simulink model "simulation_19a_lissajous"  (R2019b)
settings: Solver=VariableStepAuto  StartTime=0.0  StopTime=60  FixedStep=1e-1  RelTol=1e-3
undefined symbols (not defined in the file or in its folder): a1, a2, int_a_err, Ke, Kk, q_0
settings Model: Creator=Mathew  LastModifiedBy=Mardok
settings SFSimCC: CustomCodeUndefinedFunction=UseInterfaceOnly

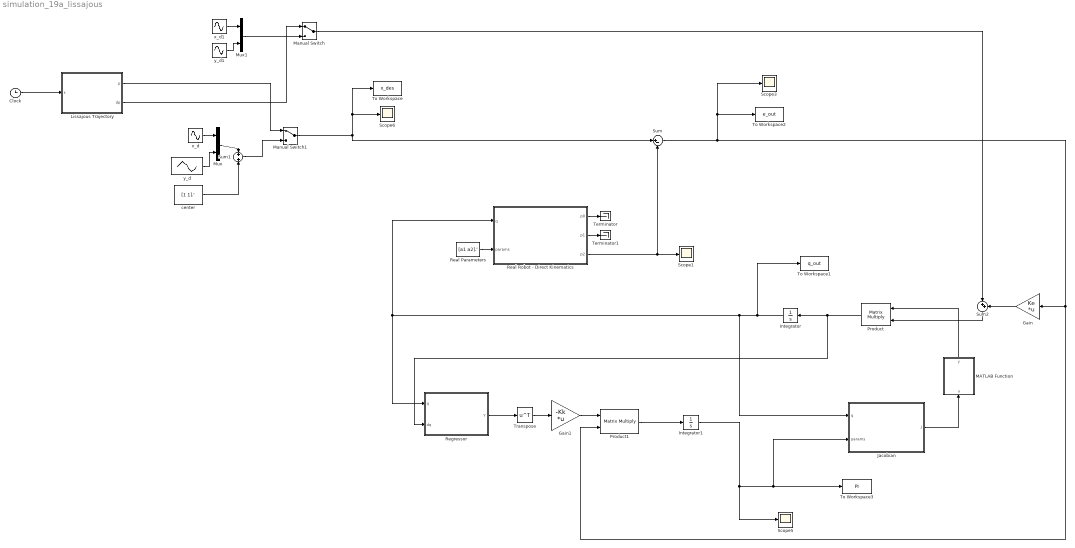
== system simulation_19a_lissajous ==
  Clock : Clock
  Gain : Gain  Gain=Ke  Multiplication=Matrix(K*u)
  Gain1 : Gain  Gain=-Kk  Multiplication=Matrix(K*u)
  Integrator : Integrator  InitialCondition=q_0
  Integrator1 : Integrator  InitialCondition=int_a_err*[a1 a2].'
  "Jacobian " : MATLAB Function  TreatAsAtomicUnit=on
  Lissajous Trajectory : MATLAB Function  TreatAsAtomicUnit=on
  MATLAB Function : MATLAB Function  TreatAsAtomicUnit=on
  Manual Switch : ManualSwitch
  Manual Switch1 : ManualSwitch
  Mux : Mux  Inputs=2
  Mux1 : Mux  Inputs=2
  Product : Product  Multiplication=Matrix(*)
  Product1 : Product  Multiplication=Matrix(*)
  Real Parameters : Constant  Value=[a1 a2].'
  Real Robot - Direct Kinematics : MATLAB Function  TreatAsAtomicUnit=on
  Regressor : MATLAB Function  TreatAsAtomicUnit=on
  Scope{1,3,5..6} (4 alike) : Scope
  Sum : Sum  Inputs=|+-
  Sum1 : Sum
  Sum2 : Sum  Inputs=|++
  Terminator : Terminator
  Terminator1 : Terminator
  To Workspace : ToWorkspace  VariableName=x_des  SaveFormat=Timeseries  SampleTime=-1
  To Workspace1 : ToWorkspace  VariableName=q_out  SaveFormat=Timeseries  SampleTime=-1
  To Workspace2 : ToWorkspace  VariableName=e_out  SaveFormat=Timeseries  SampleTime=-1
  To Workspace3 : ToWorkspace  VariableName=PI  SaveFormat=Timeseries  SampleTime=-1
  Transpose : Math  Operator=transpose  SaturateOnIntegerOverflow=on
  center : Constant  Value=[1 1].'
  x_d : Sin  Amplitude=0.25  SampleTime=0
  x_d1 : Sin  Amplitude=0.25  Phase=pi/2  SampleTime=0
  y_d : Sin  Amplitude=0.25  Phase=pi/2  SampleTime=0
  y_d1 : Sin  Amplitude=-0.25  SampleTime=0
  wires:
  Real Robot - Direct Kinematics/1(p0) -> Terminator/1
  Real Robot - Direct Kinematics/2(p1) -> Terminator1/1
  x_d/1 -> Mux/1
  y_d/1 -> Mux/2
  Manual Switch1/1 -> To Workspace/1, Scope6/1, Sum/1
  Real Robot - Direct Kinematics/3(p2) -> Scope1/1, Sum/2
  Sum/1 -> To Workspace2/1, Scope3/1, Product1/2, Gain/1
  Gain/1 -> Sum2/2
  Sum2/1 -> Product/2
  "Jacobian "/1(J) -> MATLAB Function/1(u)
  MATLAB Function/1(y) -> Product/1
  Product/1 -> Integrator/1, Regressor/2(dq)
  Integrator/1 -> To Workspace1/1, Real Robot - Direct Kinematics/1(q), Regressor/1(q), "Jacobian "/1(q)
  Regressor/1(Y) -> Transpose/1
  Transpose/1 -> Gain1/1
  Real Parameters/1 -> Real Robot - Direct Kinematics/2(params)
  Gain1/1 -> Product1/1
  Product1/1 -> Integrator1/1
  Integrator1/1 -> Scope5/1, To Workspace3/1, "Jacobian "/2(params)
  center/1 -> Sum1/2
  Mux/1 -> Sum1/1
  Manual Switch/1 -> Sum2/1
  y_d1/1 -> Mux1/2
  x_d1/1 -> Mux1/1
  Clock/1 -> Lissajous Trajectory/1(t)
  Mux1/1 -> Manual Switch/2
  Sum1/1 -> Manual Switch1/2
  Lissajous Trajectory/1(p) -> Manual Switch1/1
  Lissajous Trajectory/2(dp) -> Manual Switch/1

== matlab function simulation_19a_lissajous/Jacobian  ==
  data: q input; J output; params input
function J = J_fun( q , params)

q1 = q(1);
q2 = q(2);

a1 = params(1);
a2 = params(2);

J = [ - a2*sin(q1 + q2) - a1*sin(q1), -a2*sin(q1 + q2);
      a2*cos(q1 + q2) + a1*cos(q1),  a2*cos(q1 + q2)];

end

== matlab function simulation_19a_lissajous/Real Robot - Direct Kinematics ==
  data: q input; p0 output; params input; p1 output; p2 output
function [p0, p1, p2] = direct_kinematics(q,params)

    q1 = q(1);
    q2 = q(2);

    a1 = params(1);
    a2 = params(2);

    p0 = [0;0];
    p1 = [a1*cos(q1); a1*sin(q1)];
    p2 = p1 + [a2*cos(q1+q2); a2*sin(q1+q2)];
end

== matlab function simulation_19a_lissajous/Regressor ==
  data: q input; Y output; dq input
function Y = Y_fun( q , dq)

q1 = q(1);
q2 = q(2);
dq1 = dq(1);
dq2 = dq(2);

Y =  [ - dq1*sin(q1) , -dq1*sin(q1 + q2) - dq2*sin(q1 + q2);
         dq1*cos(q1) , dq1*cos(q1 + q2) + dq2*cos(q1 + q2) ];

end

== matlab function simulation_19a_lissajous/MATLAB Function ==
  data: u input; y output
function y = mat_inverse(u)

y = inv(u);

== matlab function simulation_19a_lissajous/Lissajous Trajectory ==
  data: t input; p output; dp output
function [p, dp] = lissajous(t)

% p0 = [1; 1];
%Optimum parameters
% A = 0.9093;
% a = 1.8929;
% d = 1.5494;
% B = 1.1402;
% b = 0.9379;

%bad trajectory
A = 1.5; B = 1;
a = -1; b = -1; d = pi;

p = [A*sin(a*t+d); B*sin(b*t)]; %+ p0;
dp = [A*a*cos(a*t+d); B*b*cos(b*t)];
